simulink model "chap1_4"  (Simulink 6.3)
settings: Solver=ode45  StartTime=0.0  StopTime=5  RelTol=1e-3
libraries: simulink x1, simulink_extras x1
settings Model: LastModifiedBy=Administrator  ExtModeTrigMode=oneshot  ExtModeArmWhenConnect=off  StrictBusMsg=None
settings DataIOCC: LimitDataPoints=off
settings OptimizationCC: BlockReduction=off  BooleanDataType=off
settings DebuggingCC: SolverPrmCheckMsg=none
settings HardwareCC: TargetUnknown=on

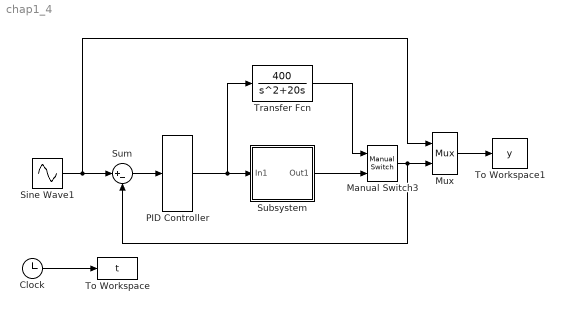
== system chap1_4 ==
  Clock : Clock
      settings: Decimation=10
  Manual Switch3 : simulink/Signal Routing/Manual Switch  sw=0  action=0
  Mux : Mux  Inputs=2
  PID Controller : simulink_extras/Additional Linear/PID Controller  P=10  I=0  D=1
  Sine Wave1 : Sin  Amplitude=0.50  Frequency=1*2*pi  SampleTime=0
  Subsystem : Subsystem
  Sum : Sum  Inputs=|+-  SaturateOnIntegerOverflow=on  InputSameDT=on
  To Workspace : ToWorkspace  VariableName=t  SampleTime=-1  SaveFormat=Array
  To Workspace1 : ToWorkspace  VariableName=y  SampleTime=-1  SaveFormat=Array
  Transfer Fcn : TransferFcn  Numerator=[400]  Denominator=[1 20 0]
  wires:
  Sum/1 -> PID Controller/1
  Sine Wave1/1 -> Sum/1, Mux/1
  Mux/1 -> To Workspace1/1
  Subsystem/1(Out1) -> Manual Switch3/2
  Transfer Fcn/1 -> Manual Switch3/1
  PID Controller/1 -> Subsystem/1(In1), Transfer Fcn/1
  Manual Switch3/1 -> Mux/2, Sum/2
  Clock/1 -> To Workspace/1

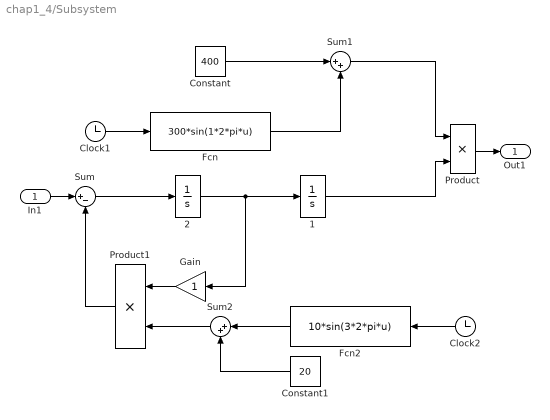
== system chap1_4/Subsystem ==
  In1 : Inport
  " 1" : Integrator
  " 2" : Integrator
  Clock1 : Clock
  Clock2 : Clock
  Constant : Constant  Value=400
  Constant1 : Constant  Orientation=left  Value=20
  "Fcn " : Fcn  Expr=300*sin(1*2*pi*u)
  Fcn2 : Fcn  Orientation=left  Expr=10*sin(3*2*pi*u)
  Gain : Gain  Orientation=left  SaturateOnIntegerOverflow=on
  Product : Product  SaturateOnIntegerOverflow=on  RndMeth=Zero  InputSameDT=on
  Product1 : Product  Orientation=left  SaturateOnIntegerOverflow=on  RndMeth=Zero  InputSameDT=on
  Sum : Sum  Inputs=|+-  SaturateOnIntegerOverflow=on  InputSameDT=on
  Sum1 : Sum  Inputs=|++  SaturateOnIntegerOverflow=on  InputSameDT=on
  Sum2 : Sum  Orientation=left  Inputs=|++  SaturateOnIntegerOverflow=on  InputSameDT=on
  Out1 : Outport
  wires:
  Sum/1 -> " 2"/1
  Clock1/1 -> "Fcn "/1
  " 1"/1 -> Product/2
  " 2"/1 -> " 1"/1, Gain/1
  Clock2/1 -> Fcn2/1
  Gain/1 -> Product1/1
  Product1/1 -> Sum/2
  Product/1 -> Out1/1
  In1/1 -> Sum/1
  "Fcn "/1 -> Sum1/2
  Constant/1 -> Sum1/1
  Sum1/1 -> Product/1
  Fcn2/1 -> Sum2/1
  Sum2/1 -> Product1/2
  Constant1/1 -> Sum2/2
